simulink model "IndustrialMicrogrid"  (R2023a)
settings: Solver=FixedStepDiscrete  StartTime=0.0  StopTime=10  FixedStep=Ts  RelTol=1e-3
PostLoadFcn:
  | IndustrialMicrogridInputData
  | GfmGridFormingConverterInputParameters
model workspace (MAT data in the model file):
  caseNum = 2
undefined symbols (not defined in the file): base, BESS, DiscIntNeverNeededParam, grid, Grid, gridInverter, machine, microgrid, PV, PVInverter, PVTransformer, scrFactorRg, scrFactorXg, transformer, Ts
libraries: ee_lib x112, eeGeneralControl x104, nesl_utility_internal x64, simulink x56, nesl_utility x37, fl_lib x29, slpidlib x13, eeTransforms x11, eeTotalHarmonicDistorsion x8, eeRmsMeasurement x4, eeSinusoidalMeasurement x4, simulink_extras x2
(part 9 of 14)

== system IndustrialMicrogrid/MG2 PV Plant/(500KWp PV)/PV Inverter A2/PV & Inverter/Measurement1 ==
  u : Inport
  Lead-Lag (Discrete or Continuous) : eeGeneralControl/Lead-Lag (Discrete or Continuous)  T1=0  T2=PV.controllerTSensor  B=inf  A=-inf  init_option=Inherited from block input  x0=0  Ts=Ts
      settings: LibrarySourceBlock=|
      | ee_sl_lib/General Control/Lead-Lag
      | (Discrete or Continuous)
  Out1 : Outport
  wires:
  u/1 -> Lead-Lag (Discrete or Continuous)/1
  Lead-Lag (Discrete or Continuous)/1 -> Out1/1

== system IndustrialMicrogrid/MG2 PV Plant/(500KWp PV)/PV Inverter A2/PV & Inverter/Measurement2 ==
  u : Inport
  Lead-Lag (Discrete or Continuous) : eeGeneralControl/Lead-Lag (Discrete or Continuous)  T1=0  T2=PV.controllerTSensor  B=inf  A=-inf  init_option=Inherited from block input  x0=0  Ts=Ts
      settings: LibrarySourceBlock=|
      | ee_sl_lib/General Control/Lead-Lag
      | (Discrete or Continuous)
  Out1 : Outport
  wires:
  u/1 -> Lead-Lag (Discrete or Continuous)/1
  Lead-Lag (Discrete or Continuous)/1 -> Out1/1

== system IndustrialMicrogrid/MG2 PV Plant/(500KWp PV)/PV Inverter A2/PV & Inverter/P&O MPP ==
  In1 : Inport
  Input : Inport  Port=2
  AND1 : Logic  IconShape=distinctive  AllPortsSameDT=off  OutDataTypeStr=boolean
  Add : Sum
  Compare To Zero1 : simulink/Logic and Bit Operations/Compare To Zero  relop=>=  OutDataTypeStr=boolean
  Compare To Zero2 : simulink/Logic and Bit Operations/Compare To Zero  relop=>=  OutDataTypeStr=boolean
  Constant1 : Constant  Value=PV.mppDv
  NOR : Logic  Operator=NOR  IconShape=distinctive  AllPortsSameDT=off  OutDataTypeStr=boolean
  OR : Logic  Operator=OR  IconShape=distinctive  AllPortsSameDT=off  OutDataTypeStr=boolean
  Subtract5 : Sum  Inputs=-+
  Sum : Sum  Inputs=|+-
  Sum1 : Sum  Inputs=|-+
  Switch4 : Switch  Criteria=u2 ~= 0  SaturateOnIntegerOverflow=off  InputSameDT=off
  Switch5 : Switch  Criteria=u2 > Threshold  SaturateOnIntegerOverflow=off  InputSameDT=off
  Unit Delay : UnitDelay  InitialCondition=2.5e5  SampleTime=PV.mppTs  HasFrameUpgradeWarning=on
  Unit Delay1 : UnitDelay  InitialCondition=1*PVInverter.Vdc  SampleTime=PV.mppTs  HasFrameUpgradeWarning=on
  ZOH/3 : ZeroOrderHold  SampleTime=0.02
  start MPPT Voltage : Constant  Value=PVInverter.Vdc  SampleTime=Ts
  Vmpp : Outport  VectorParamsAs1DForOutWhenUnconnected=off
  wires:
  [Vinc] -> Switch4/1
  ZOH/3/1 -> Vmpp/1
  Unit Delay/1 -> Sum/2
  AND1/1 -> OR/1
  Sum/1 -> Compare To Zero2/1
  Sum1/1 -> Compare To Zero1/1
  Switch4/1 -> ZOH/3/1
  [Vdec] -> Switch4/3
  Subtract5/1 -> [Vdec]  "DEC"
  NOR/1 -> OR/2
  Add/1 -> [Vinc]  "INC"
  Unit Delay1/1 -> Sum1/1
  Input/1 -> Unit Delay1/1, Sum1/2, Switch5/1, Switch5/2
  Constant1/1 -> Subtract5/1, Add/2
  Switch5/1 -> Subtract5/2, Add/1
  In1/1 -> Sum/1, Unit Delay/1
  Compare To Zero2/1 -> AND1/1, NOR/2
  start MPPT Voltage/1 -> Switch5/3
  Compare To Zero1/1 -> AND1/2, NOR/1
  OR/1 -> Switch4/2

== system IndustrialMicrogrid/MG2 PV Plant/(500KWp PV)/PV Inverter A2/PV Controller/Current_controller ==
  id-ref : Inport
  ipvd : Inport  Port=2
  iqref : Inport  Port=3
  iq : Inport  Port=4
  Vd : Inport  Port=5
  Vq : Inport  Port=6
  Constant4 : Constant  Value=0
  Gain1 : Gain  Gain=2*1*pi*60*PVInverter.l/PV.zBase
  Gain2 : Gain  Gain=2*1*pi*60*PVInverter.l/PV.zBase
  Mux1 : Mux  Inputs=3
  PID Controller : slpidlib/PID Controller  Controller=PID  Form=Parallel  TimeDomain=Discrete-time  UseExternalTs=off  SampleTime=-1  IntegratorMethod=Forward Euler  FilterMethod=Forward Euler  ControllerParametersSource=internal  P=PV.controllerKpIc*0.02*2  I=PV.controllerKiIc*0.02*2  UseKiTs=off  D=PV.controllerKd  N=100  UseFilter=off  TunerSelectOption=Transfer Function Based (PID Tuner App)  InitialConditionSource=internal  InitialConditionForIntegrator=-0.023  InitialConditionForFilter=0  DifferentiatorICPrevScaledInput=0  ExternalReset=none  TrackingMode=off  Kt=1  LimitOutput=off  SatLimitsSource=internal  UpperSaturationLimit=1.5  LowerSaturationLimit=-1.5  LinearizeAsGain=on  AntiWindupMode=clamping  Kb=1  LimitIntegrator=off  UpperIntegratorSaturationLimit=1.5  LowerIntegratorSaturationLimit=-1.5  POutMin=[]  POutMax=[]  IOutMin=[]  IOutMax=[]  DOutMin=[]  DOutMax=[]  NOutMin=[]  NOutMax=[]  SumOutMin=[]  SumOutMax=[]  SaturationOutMin=[]  SaturationOutMax=[]  PParamMin=[]  PParamMax=[]  IParamMin=[]  IParamMax=[]  DParamMin=[]  DParamMax=[]  NParamMin=[]  NParamMax=[]  KbParamMin=[]  KbParamMax=[]  KtParamMin=[]  KtParamMax=[]  KbOutMin=[]  KbOutMax=[]  KtOutMin=[]  KtOutMax=[]  IntegratorOutMin=[]  IntegratorOutMax=[]  FilterOutMin=[]  FilterOutMax=[]  SumI1OutMin=[]  SumI1OutMax=[]  SumI2OutMin=[]  SumI2OutMax=[]  SumI3OutMin=[]  SumI3OutMax=[]  SumI4OutMin=[]  SumI4OutMax=[]  SumDOutMin=[]  SumDOutMax=[]  DifferentiatorOutMin=[]  DifferentiatorOutMax=[]  FilterDiffOutCoefMin=[]  FilterDiffOutCoefMax=[]  ReciprocalOutMin=[]  ReciprocalOutMax=[]  SumDenOutMin=[]  SumDenOutMax=[]  SumNumOutMin=[]  SumNumOutMax=[]  DivideOutMin=[]  DivideOutMax=[]  UdiffTsProdOutMin=[]  UdiffTsProdOutMax=[]  NTsProdOutMin=[]  NTsProdOutMax=[]  UintegralTsProdOutMin=[]  UintegralTsProdOutMax=[]  UngainTsProdOutMin=[]  UngainTsProdOutMax=[]  ClampingZeroOutDataTypeStr=Inherit: Inherit via back propagation  ClampingZeroOutMin=[]  ClampingZeroOutMax=[]  FilterDenConstantOutDataTypeStr=Inherit: Inherit via back propagation  FilterDenConstantOutMin=[]  FilterDenConstantOutMax=[]  PCopyOutDataTypeStr=Inherit: Inherit via back propagation  PCopyOutMin=[]  PCopyOutMax=[]  NCopyOutDataTypeStr=Inherit: Inherit via back propagation  NCopyOutMin=[]  NCopyOutMax=[]  IntegratorContinuousStateAttributes=''  IntegratorStateMustResolveToSignalObject=off  IntegratorRTWStateStorageClass=Auto  FilterContinuousStateAttributes=''  FilterStateMustResolveToSignalObject=off  FilterRTWStateStorageClass=Auto  ParallelPVariant=InternalParameters  IdealPVariant=Disabled  IVariant=InternalParameters  DVariant=InternalParameters  IntegratorVariant=Discrete  SatVariant=Disabled  AWVariant=Passthrough  PCopyVariant=Disabled  TRVariant=Disabled  FdbkBlocksVariant=Forward  IdealPFdbkVariant=Disabled  SatFdbkVariant=Disabled  DerivativeFilterVariant=Differentiator  NVariant=Passthrough  NCopyVariant=Disabled_SignalSpec  FilterICVariant=InternalICsDifferentiator  IntegratorICVariant=InternalICs  ExternalResetVariant=Disabled  TRSumVariant=Passthrough  SumFdbkVariant=Disabled  SumVariant=Sum_PID  TsampFilterVariant=InternalTs  TsampNgainVariant=Passthrough  TsampIntegralVariant=Disabled_SignalSpec  ExternalSaturationOutDataTypeStr=Inherit: Same as second input
  PID Controller1 : slpidlib/PID Controller  Controller=PID  Form=Parallel  TimeDomain=Discrete-time  UseExternalTs=off  SampleTime=-1  IntegratorMethod=Forward Euler  FilterMethod=Forward Euler  ControllerParametersSource=internal  P=PV.controllerKpIc*10  I=PV.controllerKiIc*0.2  UseKiTs=off  D=PV.controllerKd  N=100  UseFilter=off  TunerSelectOption=Transfer Function Based (PID Tuner App)  InitialConditionSource=internal  InitialConditionForIntegrator=0.4  InitialConditionForFilter=0  DifferentiatorICPrevScaledInput=0  ExternalReset=none  TrackingMode=off  Kt=1  LimitOutput=off  SatLimitsSource=internal  UpperSaturationLimit=1.5  LowerSaturationLimit=-1.5  LinearizeAsGain=on  AntiWindupMode=clamping  Kb=1  LimitIntegrator=off  UpperIntegratorSaturationLimit=1.5  LowerIntegratorSaturationLimit=-1.5  POutMin=[]  POutMax=[]  IOutMin=[]  IOutMax=[]  DOutMin=[]  DOutMax=[]  NOutMin=[]  NOutMax=[]  SumOutMin=[]  SumOutMax=[]  SaturationOutMin=[]  SaturationOutMax=[]  PParamMin=[]  PParamMax=[]  IParamMin=[]  IParamMax=[]  DParamMin=[]  DParamMax=[]  NParamMin=[]  NParamMax=[]  KbParamMin=[]  KbParamMax=[]  KtParamMin=[]  KtParamMax=[]  KbOutMin=[]  KbOutMax=[]  KtOutMin=[]  KtOutMax=[]  IntegratorOutMin=[]  IntegratorOutMax=[]  FilterOutMin=[]  FilterOutMax=[]  SumI1OutMin=[]  SumI1OutMax=[]  SumI2OutMin=[]  SumI2OutMax=[]  SumI3OutMin=[]  SumI3OutMax=[]  SumI4OutMin=[]  SumI4OutMax=[]  SumDOutMin=[]  SumDOutMax=[]  DifferentiatorOutMin=[]  DifferentiatorOutMax=[]  FilterDiffOutCoefMin=[]  FilterDiffOutCoefMax=[]  ReciprocalOutMin=[]  ReciprocalOutMax=[]  SumDenOutMin=[]  SumDenOutMax=[]  SumNumOutMin=[]  SumNumOutMax=[]  DivideOutMin=[]  DivideOutMax=[]  UdiffTsProdOutMin=[]  UdiffTsProdOutMax=[]  NTsProdOutMin=[]  NTsProdOutMax=[]  UintegralTsProdOutMin=[]  UintegralTsProdOutMax=[]  UngainTsProdOutMin=[]  UngainTsProdOutMax=[]  ClampingZeroOutDataTypeStr=Inherit: Inherit via back propagation  ClampingZeroOutMin=[]  ClampingZeroOutMax=[]  FilterDenConstantOutDataTypeStr=Inherit: Inherit via back propagation  FilterDenConstantOutMin=[]  FilterDenConstantOutMax=[]  PCopyOutDataTypeStr=Inherit: Inherit via back propagation  PCopyOutMin=[]  PCopyOutMax=[]  NCopyOutDataTypeStr=Inherit: Inherit via back propagation  NCopyOutMin=[]  NCopyOutMax=[]  IntegratorContinuousStateAttributes=''  IntegratorStateMustResolveToSignalObject=off  IntegratorRTWStateStorageClass=Auto  FilterContinuousStateAttributes=''  FilterStateMustResolveToSignalObject=off  FilterRTWStateStorageClass=Auto  ParallelPVariant=InternalParameters  IdealPVariant=Disabled  IVariant=InternalParameters  DVariant=InternalParameters  IntegratorVariant=Discrete  SatVariant=Disabled  AWVariant=Passthrough  PCopyVariant=Disabled  TRVariant=Disabled  FdbkBlocksVariant=Forward  IdealPFdbkVariant=Disabled  SatFdbkVariant=Disabled  DerivativeFilterVariant=Differentiator  NVariant=Passthrough  NCopyVariant=Disabled_SignalSpec  FilterICVariant=InternalICsDifferentiator  IntegratorICVariant=InternalICs  ExternalResetVariant=Disabled  TRSumVariant=Passthrough  SumFdbkVariant=Disabled  SumVariant=Sum_PID  TsampFilterVariant=InternalTs  TsampNgainVariant=Passthrough  TsampIntegralVariant=Disabled_SignalSpec  ExternalSaturationOutDataTypeStr=Inherit: Same as second input
  Sum1 : Sum  Inputs=|+-
  Sum3 : Sum  Inputs=|++-
  Sum4 : Sum  Inputs=|+++
  Sum5 : Sum  Inputs=|+-
  Refrence_mdq0 : Outport
  wires:
  ipvd/1 -> Sum1/2, Gain1/1
  id-ref/1 -> Sum1/1
  iq/1 -> Sum5/2, Gain2/1
  iqref/1 -> Sum5/1
  Vd/1 -> Sum3/1
  Vq/1 -> Sum4/2
  Mux1/1 -> Refrence_mdq0/1  "m_dqo"
  Sum4/1 -> Mux1/2
  PID Controller1/1 -> Sum4/1
  Sum5/1 -> PID Controller1/1
  Constant4/1 -> Mux1/3
  Sum1/1 -> PID Controller/1
  Gain1/1 -> Sum4/3
  Gain2/1 -> Sum3/3
  Sum3/1 -> Mux1/1
  PID Controller/1 -> Sum3/2

== system IndustrialMicrogrid/MG2 PV Plant/(500KWp PV)/PV Inverter A2/PV Controller/DC voltage controller & current reference ==
  note: id_ref_generator
  note: iq_ref_generator
  note: Limiter
  Q_ref : Inport
  Vmag : Inport  Port=2
  P_pv : Inport  Port=3
  PV_Mpp_vdc : Inport  Port=4
  PV_vdc : Inport  Port=5
  LVRT.iq : Inport  Port=6
  Constant : Constant
  Constant1 : Constant  Value=PVInverter.iMaxPU
  Current limits : Subsystem
  Subsystem : Subsystem
  Subsystem1 : Subsystem
  Switch : Switch  Criteria=u2 > Threshold  SaturateOnIntegerOverflow=off  InputSameDT=off
  Unit Delay1 : UnitDelay  SampleTime=Ts  HasFrameUpgradeWarning=on
  Unit Delay3 : UnitDelay  SampleTime=Ts  HasFrameUpgradeWarning=on
  iq_ref : Outport
  id_ref : Outport  Port=2
  wires:
  Constant/1 -> Switch/3
  Switch/1 -> Subsystem1/1(Vmag), Subsystem/1(V_mag)
  Vmag/1 -> Switch/1, Switch/2
  LVRT.iq/1 -> Subsystem/3(LVRT.iq)
  [ubiq] -> Subsystem/2(iq_ub)
  [ubid] -> Subsystem1/5(id_ub)
  Subsystem/1(Out1) -> iq_ref/1, [iq_ref]
  PV_vdc/1 -> Subsystem1/4(PV_vdc)
  PV_Mpp_vdc/1 -> Subsystem1/3(PV_Mpp_vdc)
  P_pv/1 -> Subsystem1/2(P_pv)
  Subsystem1/1(Out1) -> id_ref/1, [id_ref]
  Q_ref/1 -> Subsystem/4(Q_ref)
  Unit Delay3/1 -> Current limits/3(idref)
  [id_ref] -> Unit Delay3/1
  Unit Delay1/1 -> Current limits/2(iqref)
  Constant1/1 -> Current limits/1(Imax)
  Current limits/1(iubd) -> [ubid]
  Current limits/2(iubq) -> [ubiq]
  [iq_ref] -> Unit Delay1/1

== system IndustrialMicrogrid/MG2 Primary Substation/BESS and Controller 2/BESS/Grid-Forming Converter Control/Current Limiting ==
  In Bus Element : Inport  PortName=measure  Element=Igd
  In Bus Element1 : Inport  PortName=measure  Element=Igq
  In Bus Element2 : Inport  Port=2  PortName=reactiveControl  Element=Vmd
  In Bus Element4 : Inport  Port=2  PortName=reactiveControl  Element=Vmq
  CurrentLimitingMethod : Subsystem  Variant=on  VariantControlMode=label  VariantControl=Choice  LabelModeActiveChoice=virimp
  Subtract : Sum  Inputs=+-
  Subtract1 : Sum  Inputs=-+
  Out Bus Element : Outport  PortName=currentLimiting  Element=Vmd
  Out Bus Element1 : Outport  PortName=currentLimiting  Element=Vmq
  Out Bus Element2 : Outport  PortName=currentLimiting  Element=Idmax
  Out Bus Element3 : Outport  PortName=currentLimiting  Element=Iqmax
  wires:
  In Bus Element2/1 -> Subtract/1
  In Bus Element1/1 -> CurrentLimitingMethod/2(Igq)
  In Bus Element4/1 -> Subtract1/2
  Subtract/1 -> Out Bus Element/1
  Subtract1/1 -> Out Bus Element1/1
  CurrentLimitingMethod/4(Iqmax) -> Out Bus Element3/1
  In Bus Element/1 -> CurrentLimitingMethod/1(Igd)  "Q"
  CurrentLimitingMethod/3(Idmax) -> Out Bus Element2/1
  CurrentLimitingMethod/1(delVd) -> Subtract/2
  CurrentLimitingMethod/2(delVq) -> Subtract1/1

== system IndustrialMicrogrid/MG2 Primary Substation/BESS and Controller 2/BESS/Grid-Forming Converter Control/Grid Voltage Reactive Power Support ==
  In Bus Element1 : Inport  PortName=measure  Element=Vgd
  In Bus Element3 : Inport  PortName=measure  Element=Vgq
  In Bus Element2 : Inport  PortName=measure  Element=Igd
  In Bus Element4 : Inport  PortName=measure  Element=Igq
  PrefInput : Inport  Port=2
  QrefInput : Inport  Port=3
  Modifying Active Power Reference : Subsystem
  Modifying Reactive Power Reference : Subsystem
  Pref : Outport
  Qref : Outport  Port=2
  wires:
  Modifying Active Power Reference/1(Pref) -> Modifying Reactive Power Reference/4(Pref)
  PrefInput/1 -> Modifying Active Power Reference/1(PrefInput)
  In Bus Element2/1 -> Modifying Active Power Reference/3(Igd)
  In Bus Element4/1 -> Modifying Active Power Reference/4(Igq)
  In Bus Element1/1 -> Modifying Reactive Power Reference/1(Vgd), Modifying Active Power Reference/2(Vd)
  In Bus Element3/1 -> Modifying Reactive Power Reference/2(Vgq)
  QrefInput/1 -> Modifying Reactive Power Reference/3(Qref)
  Modifying Reactive Power Reference/1(PrefNew) -> Pref/1
  Modifying Reactive Power Reference/2(QrefNew) -> Qref/1

== system IndustrialMicrogrid/MG2 Primary Substation/BESS and Controller 2/BESS/Grid-Forming Converter Control/Measurement ==
  Vgabcc : Inport
  Igabc : Inport  Port=2
  Angle : Inport  Port=3
  Frequency Measurement : Subsystem
  Gain1 : Gain  Gain=1/power
  Gain2 : Gain  Gain=1/power
  Gain3 : Gain  Gain=1/(girdLineVoltage*sqrt(2/3))
  Gain4 : Gain  Gain=1/(girdLineVoltage*sqrt(2/3))
  Gain5 : Gain  Gain=1/(power/(sqrt(3)*girdLineVoltage)*sqrt(2))
  Gain6 : Gain  Gain=1/(power/(sqrt(3)*girdLineVoltage)*sqrt(2))
  Power Measurement (Three-Phase) : eePowerMeasurement/Power Measurement (Three-Phase)  LabelModeActiveChoice=Discrete  F=powerFreq  K=[1]  Seq=Positive  Ts=measSampleTime
  abc2dq : Subsystem
  Out Bus Element : Outport  PortName=measure  Element=P
  Out Bus Element1 : Outport  PortName=measure  Element=Q
  Out Bus Element2 : Outport  PortName=measure  Element=Vgd
  Out Bus Element3 : Outport  PortName=measure  Element=Vgq
  Out Bus Element4 : Outport  PortName=measure  Element=Igd
  Out Bus Element5 : Outport  PortName=measure  Element=Igq
  Out Bus Element6 : Outport  PortName=measure  Element=fgrid
  Pmeas : Outport  Port=2
  Qmeas : Outport  Port=3
  fmeas : Outport  Port=4
  wires:
  Vgabcc/1 -> abc2dq/3(Vgabc), Frequency Measurement/1(Vabc), Power Measurement (Three-Phase)/1  "Vabc"
  Angle/1 -> abc2dq/2(Angle)
  Power Measurement (Three-Phase)/1 -> Gain2/1
  Igabc/1 -> abc2dq/1(Igabc), Power Measurement (Three-Phase)/2  "Iabc"
  Power Measurement (Three-Phase)/2 -> Gain1/1
  Gain2/1 -> Pmeas/1, Out Bus Element/1  "Pmeas"
  Gain1/1 -> Qmeas/1, Out Bus Element1/1  "Qmeas"
  abc2dq/1(Vgd) -> Gain4/1
  abc2dq/2(Vgq) -> Gain3/1
  abc2dq/3(Igd) -> Gain5/1
  abc2dq/4(Igq) -> Gain6/1
  Gain3/1 -> Out Bus Element3/1  "Vgq"
  Gain4/1 -> Out Bus Element2/1  "Vgd"
  Gain5/1 -> Out Bus Element4/1  "Igd"
  Gain6/1 -> Out Bus Element5/1  "Igq"
  Frequency Measurement/1(freq) -> Out Bus Element6/1, fmeas/1

== system IndustrialMicrogrid/MG2 Primary Substation/BESS and Controller 2/BESS/Grid-Forming Converter Control/Power Control ==
  note: Reactive Power Control
  note: Active Power Control
  In Bus Element2 : Inport  PortName=measure  Element=P
  In Bus Element1 : Inport  PortName=measure  Element=fgrid
  BusElementIn : Inport  PortName=measure  Element=Vgd
  BusElementIn2 : Inport  PortName=measure  Element=Q
  Pref : Inport  Port=2
  Qref : Inport  Port=3
  Vref : Inport  Port=4
  Fref : Inport  Port=5
  CntrlFlag : Inport  Port=6
  ActivePowerControl : Subsystem  Variant=on  VariantControlMode=label  VariantControl=Choice  LabelModeActiveChoice=vsm
  ReactiveControl : Subsystem
  Scope : Scope
  Out Bus Element : Outport  PortName=reactiveControl  Element=Vmd
  Out Bus Element1 : Outport  PortName=reactiveControl  Element=Vmq
  Out Bus Element6 : Outport  Port=2  PortName=activeControl  Element=angle
  Out Bus Element4 : Outport  Port=2  PortName=activeControl  Element=w
  angle : Outport  Port=3
  wires:
  ActivePowerControl/2(w) -> Out Bus Element4/1
  ActivePowerControl/1(Theta) -> angle/1, Out Bus Element6/1
  ReactiveControl/1(Vmd) -> Out Bus Element/1
  ReactiveControl/2(Vmq) -> Out Bus Element1/1
  Pref/1 -> ActivePowerControl/1(Pref)  "Q"
  Qref/1 -> ReactiveControl/2(Qref)  "Q"
  In Bus Element2/1 -> ActivePowerControl/2(Pmeas)
  In Bus Element1/1 -> ActivePowerControl/5(fgrid)
  Fref/1 -> ActivePowerControl/3(fref)
  CntrlFlag/1 -> [Cntrlflag]
  [Cntrlflag] -> ActivePowerControl/4(cntrlflag)
  Vref/1 -> ReactiveControl/5(Vref)
  [Cntrlflag] -> ReactiveControl/1(CntrlFlag)
  BusElementIn/1 -> Scope/1, ReactiveControl/4(Vgdmeas)
  BusElementIn2/1 -> ReactiveControl/3(Qmeas)

== system IndustrialMicrogrid/MG2 Primary Substation/BESS and Controller 2/BESS/Grid-Forming Converter Control/VoltageCurrentControl ==
  In Bus Element : Inport  PortName=currentLimiting  Element=Vmd
  In Bus Element1 : Inport  PortName=currentLimiting  Element=Vmq
  In Bus Element6 : Inport  PortName=currentLimiting  Element=Idmax
  In Bus Element7 : Inport  PortName=currentLimiting  Element=Iqmax
  Bus Element In6 : Inport  Port=2  PortName=activeControl  Element=w
  Bus Element In1 : Inport  Port=2  PortName=activeControl  Element=angle
  BlackStart : Inport  Port=3
  In Bus Element2 : Inport  Port=4  PortName=measure  Element=Vgd
  In Bus Element3 : Inport  Port=4  PortName=measure  Element=Vgq
  In Bus Element4 : Inport  Port=4  PortName=measure  Element=Igd
  In Bus Element5 : Inport  Port=4  PortName=measure  Element=Igq
  Controller : Subsystem
      settings: PortSchema="{\"entries\":[{\"content\":{\"sides\":[{\"content\":{\"connectorIds\":[\"In1\",\"In2\",\"In3\",\"In4\",\"In5\",\"In6\",\"In7\",\"In8\",\"In9\"]},\"type\":\"ConnectorPlacement.EquallySpacedRectSide\",\"uuid\":\"29d30ab3-0ae0-4ae6-aaee-46c6f5faca9c\"},{\"content\":{\"connectorIds\":[\"Out1\",\"Out2\"],\"side\":\"RIGHT\"},\"type\":\"ConnectorPlacement.EquallySpacedRectSide\",\"uuid\":\"4918c3a7-9f8f-4af5-ac25-a0a0710917b2\"},{\"content\":{\"connectorIds\":[\"In10\"],\"side\":\"TOP\"},\"type\":\"ConnectorPlacement.EquallySpacedRectSide\",\"uuid\":\"c6ee8000-0a39-46c2-b8e8-8b73a56a82d9\"}]},\"type\":\"ConnectorPlacement.EquallySpacedConnector\",\"uuid\":\"193e0bc8-3764-41d1-9278-3938c4a9e9f5\"}],\"packageUris\":[\"http://schema.mathworks.com/mf0/Connector/R2020b\"],\"version\":\"1.0\"}"
  Modulation Signal : Subsystem
  mabc : Outport
  wires:
  Controller/2(Vq) -> Modulation Signal/2(Vq)
  Modulation Signal/1(mabc) -> mabc/1
  Controller/1(Vd) -> Modulation Signal/1(Vd)
  In Bus Element4/1 -> Controller/6(Id)
  In Bus Element5/1 -> Controller/7(Iq)
  In Bus Element6/1 -> Controller/8(Idmax)
  In Bus Element7/1 -> Controller/9(Iqmax)
  In Bus Element2/1 -> Controller/4(Vsd)
  In Bus Element3/1 -> Controller/5(Vsq)
  Bus Element In6/1 -> Controller/1(Angfreq)
  In Bus Element/1 -> Controller/2(Vgdref)
  In Bus Element1/1 -> Controller/3(Vgqref)
  Bus Element In1/1 -> Modulation Signal/3(Angle)
  BlackStart/1 -> Controller/10(BlackStart1)

== system IndustrialMicrogrid/MG2 Primary Substation/Microgrid Controller 2/Black Start/If Action Subsystem/Subsystem ==
  Constant2 : Constant  DisableCoverage=on  Value=-(Controller2BlackStart+Controller2BlackStartDelay)  OutDataTypeStr=Inherit: Inherit via back propagation  SampleTime=Ts
  Digital Clock : DigitalClock  SampleTime=Ts
  Output : Sum  Inputs=|++  InputSameDT=on  SaturateOnIntegerOverflow=on  OutDataTypeStr=Inherit: Same as first input
  Product : Product  DisableCoverage=on  InputSameDT=on  SaturateOnIntegerOverflow=on  OutDataTypeStr=Inherit: Same as first input
  Saturation : Saturate  UpperLimit=Controller2BlackStartVoltageLevel1  LowerLimit=0
  Step : Step  DisableCoverage=on  Time=Controller2BlackStart+Controller2BlackStartDelay  OutDataTypeStr=fixdt('double', 'DataTypeOverride', 'Off')  SampleTime=Ts
  Out1 : Outport
  wires:
  Step/1 -> Product/1
  Output/1 -> Saturation/1
  Product/1 -> Output/1
  Saturation/1 -> Out1/1
  Constant2/1 -> Output/2
  Digital Clock/1 -> Product/2

== system IndustrialMicrogrid/MG2 Primary Substation/Microgrid Controller 2/Black Start/If Action Subsystem/Subsystem1 ==
  Constant2 : Constant  DisableCoverage=on  Value=-(Controller2BlackStart+Controller2BlackStartDelay+Controller2BlackStartDelayLevel2)  OutDataTypeStr=Inherit: Inherit via back propagation  SampleTime=Ts
  Digital Clock : DigitalClock  SampleTime=Ts
  Output : Sum  Inputs=|++  InputSameDT=on  SaturateOnIntegerOverflow=on  OutDataTypeStr=Inherit: Same as first input
  Product : Product  DisableCoverage=on  InputSameDT=on  SaturateOnIntegerOverflow=on  OutDataTypeStr=Inherit: Same as first input
  Saturation : Saturate  UpperLimit=Controller2BlackStartVoltageLevel2  LowerLimit=0
  Step : Step  DisableCoverage=on  Time=Controller2BlackStart+Controller2BlackStartDelay+Controller2BlackStartDelayLevel2  OutDataTypeStr=fixdt('double', 'DataTypeOverride', 'Off')  SampleTime=Ts
  Out1 : Outport
  wires:
  Digital Clock/1 -> Product/2
  Constant2/1 -> Output/2
  Saturation/1 -> Out1/1
  Product/1 -> Output/1
  Output/1 -> Saturation/1
  Step/1 -> Product/1

== system IndustrialMicrogrid/MG2 Primary Substation/Microgrid Controller 2/Black Start/If Action Subsystem/Subsystem2 ==
  Constant2 : Constant  DisableCoverage=on  Value=-(Controller2BlackStart+Controller2BlackStartDelay+Controller2BlackStartDelayLevel2+Controller2BlackStartDelayLevel3)  OutDataTypeStr=Inherit: Inherit via back propagation  SampleTime=Ts
  Digital Clock : DigitalClock  SampleTime=Ts
  Output : Sum  Inputs=|++  InputSameDT=on  SaturateOnIntegerOverflow=on  OutDataTypeStr=Inherit: Same as first input
  Product : Product  DisableCoverage=on  InputSameDT=on  SaturateOnIntegerOverflow=on  OutDataTypeStr=Inherit: Same as first input
  Saturation : Saturate  UpperLimit=Controller2BlackStartVoltageLevel3  LowerLimit=0
  Step : Step  DisableCoverage=on  Time=Controller2BlackStart+Controller2BlackStartDelay+Controller2BlackStartDelayLevel2+Controller2BlackStartDelayLevel3  OutDataTypeStr=fixdt('double', 'DataTypeOverride', 'Off')  SampleTime=Ts
  Out1 : Outport
  wires:
  Step/1 -> Product/1
  Output/1 -> Saturation/1
  Product/1 -> Output/1
  Saturation/1 -> Out1/1
  Constant2/1 -> Output/2
  Digital Clock/1 -> Product/2

== system IndustrialMicrogrid/MG2 Primary Substation/Microgrid Controller 2/PLL /PLL/Subsystem ==
  In : Inport
  Bias : Bias  Bias=180  SaturateOnIntegerOverflow=off
  Bias1 : Bias  Bias=-180  SaturateOnIntegerOverflow=off
  Constant : Constant  Value=grid.frequency
  Constant1 : Constant  Value=360
  Data Type Conversion Inherited : simulink/Signal Attributes/Data Type Conversion Inherited  ConvertRealWorld=Real World Value  DoSatur=off
  Digital Clock : DigitalClock  SampleTime=Ts
  Mod : Math  Operator=mod
  Product : Product
  Sum : Sum  Inputs=+-  OutDataTypeStr=Inherit: Same as first input
  gain : Gain  Gain=2*pi
  rad2deg : Gain  Gain=180/pi
  Out : Outport
  wires:
  Bias1/1 -> Out/1
  Product/1 -> Sum/2
  In/1 -> Sum/1
  gain/1 -> Product/1
  Constant/1 -> gain/1
  Bias/1 -> Mod/1
  Mod/1 -> Bias1/1
  Digital Clock/1 -> Product/2
  Constant1/1 -> Data Type Conversion Inherited/2
  rad2deg/1 -> Data Type Conversion Inherited/1, Bias/1
  Sum/1 -> rad2deg/1
  Data Type Conversion Inherited/1 -> Mod/2

== system IndustrialMicrogrid/MG2 Primary Substation/Microgrid Controller 2/PLL /PLL1/Subsystem ==
  In : Inport
  Bias : Bias  Bias=180  SaturateOnIntegerOverflow=off
  Bias1 : Bias  Bias=-180  SaturateOnIntegerOverflow=off
  Constant : Constant  Value=grid.frequency
  Constant1 : Constant  Value=360
  Data Type Conversion Inherited : simulink/Signal Attributes/Data Type Conversion Inherited  ConvertRealWorld=Real World Value  DoSatur=off
  Digital Clock : DigitalClock  SampleTime=Ts
  Mod : Math  Operator=mod
  Product : Product
  Sum : Sum  Inputs=+-  OutDataTypeStr=Inherit: Same as first input
  gain : Gain  Gain=2*pi
  rad2deg : Gain  Gain=180/pi
  Out : Outport
  wires:
  Data Type Conversion Inherited/1 -> Mod/2
  Sum/1 -> rad2deg/1
  rad2deg/1 -> Bias/1, Data Type Conversion Inherited/1
  Constant1/1 -> Data Type Conversion Inherited/2
  Digital Clock/1 -> Product/2
  Mod/1 -> Bias1/1
  Bias/1 -> Mod/1
  Constant/1 -> gain/1
  gain/1 -> Product/1
  In/1 -> Sum/1
  Product/1 -> Sum/2
  Bias1/1 -> Out/1

== system IndustrialMicrogrid/MG2 Primary Substation/Microgrid Controller 2/Planned Island/Control for Zero Powerflow1/Planned Island Time Delay ==
  In1 : Inport
  In2 : Inport  Port=2
  Cast To Double : DataTypeConversion  OutDataTypeStr=double  SaturateOnIntegerOverflow=off  RndMeth=Floor
  Constant3 : Constant  Value=0
  Delay1 : Delay  DelayLength=500  SampleTime=Ts
  Delay2 : Delay  DelayLength=PlannedIslandDelay  InitialCondition=0  SampleTime=Ts*5
  Monostable Flip-Flop : eeGeneralControl/Monostable Flip-Flop  VariantControl=Variant1  LabelModeActiveChoice=Discrete  ChangeType=Rising edge  x0=0  Td=100  Ts=Ts
      settings: LibrarySourceBlock=ee_sl_lib/General Control/Monostable Flip-Flop
  Switch : Switch  Criteria=u2 > Threshold  Threshold=0.5  SaturateOnIntegerOverflow=off  InputSameDT=off
  MGController : Outport
  wires:
  In2/1 -> Delay1/1
  In1/1 -> Switch/1
  Monostable Flip-Flop/1 -> Cast To Double/1
  Delay2/1 -> MGController/1
  Delay1/1 -> Switch/2
  Constant3/1 -> Switch/3
  Cast To Double/1 -> Delay2/1
  Switch/1 -> Monostable Flip-Flop/1

== system IndustrialMicrogrid/MG2 Primary Substation/Microgrid Controller 2/Planned Island/Control for Zero Powerflow1/Subsystem ==
  AVTIVE POWER ERROR : Inport
  AND : Logic  IconShape=distinctive  AllPortsSameDT=off  OutDataTypeStr=boolean
  Abs : Abs  SaturateOnIntegerOverflow=off
  Constant : Constant  Value=ZeroActivePowerThreshold  SampleTime=-1
  Delay : Delay  DelayLength=1000  SampleTime=Ts
  Relational Operator : RelationalOperator  Operator=<=  OutDataTypeStr=boolean  RndMeth=Simplest  InputSameDT=off
  Out1 : Outport
  wires:
  Delay/1 -> AND/2
  Constant/1 -> Relational Operator/2
  Relational Operator/1 -> AND/1, Delay/1
  AND/1 -> Out1/1
  AVTIVE POWER ERROR/1 -> Abs/1
  Abs/1 -> Relational Operator/1

== system IndustrialMicrogrid/MG2 Primary Substation/Microgrid Controller 2/Planned Island/Control for Zero Powerflow1/Subsystem1 ==
  REACTIVEPOWER ERROR : Inport
  AND : Logic  IconShape=distinctive  AllPortsSameDT=off  OutDataTypeStr=boolean
  Abs : Abs  SaturateOnIntegerOverflow=off
  Constant2 : Constant  Value=ZeroReactivePowerThreshold
  Delay : Delay  DelayLength=1000  SampleTime=Ts
  Relational Operator2 : RelationalOperator  Operator=<=  OutDataTypeStr=boolean  RndMeth=Simplest  InputSameDT=off
  Out1 : Outport
  wires:
  Delay/1 -> AND/2
  REACTIVEPOWER ERROR/1 -> Abs/1
  Relational Operator2/1 -> Delay/1, AND/1
  Constant2/1 -> Relational Operator2/2
  AND/1 -> Out1/1
  Abs/1 -> Relational Operator2/1

== system IndustrialMicrogrid/MG2 Primary Substation/Microgrid Controller 2/Resynchronization/Frequency and voltage matching/Resynchronization Time Delay ==
  In1 : Inport
  In2 : Inport  Port=2
  Cast To Double : DataTypeConversion  OutDataTypeStr=double  SaturateOnIntegerOverflow=off  RndMeth=Floor
  Constant3 : Constant  Value=0
  Delay1 : Delay  DelayLength=500  SampleTime=Ts
  Delay2 : Delay  DelayLength=ResynchDelay  InitialCondition=0  SampleTime=Ts*5
  Monostable Flip-Flop : eeGeneralControl/Monostable Flip-Flop  VariantControl=Variant1  LabelModeActiveChoice=Discrete  ChangeType=Rising edge  x0=0  Td=100  Ts=Ts
      settings: LibrarySourceBlock=ee_sl_lib/General Control/Monostable Flip-Flop
  Switch : Switch  Criteria=u2 > Threshold  Threshold=0.5  SaturateOnIntegerOverflow=off  InputSameDT=off
  MGController : Outport
  wires:
  Switch/1 -> Monostable Flip-Flop/1
  Cast To Double/1 -> Delay2/1
  Constant3/1 -> Switch/3
  Delay1/1 -> Switch/2
  Delay2/1 -> MGController/1
  Monostable Flip-Flop/1 -> Cast To Double/1
  In1/1 -> Switch/1
  In2/1 -> Delay1/1

== system IndustrialMicrogrid/MG2 Primary Substation/Microgrid Controller 2/Resynchronization/Frequency and voltage matching/Subsystem ==
  FREQUENCY ERROR : Inport
  AND : Logic  IconShape=distinctive  AllPortsSameDT=off  OutDataTypeStr=boolean
  Abs : Abs  SaturateOnIntegerOverflow=off
  Constant : Constant  Value=FrequencyThreshold  SampleTime=-1
  Delay : Delay  DelayLength=1000  SampleTime=Ts
  Relational Operator : RelationalOperator  Operator=<=  OutDataTypeStr=boolean  RndMeth=Simplest  InputSameDT=off
  Out1 : Outport
  wires:
  Delay/1 -> AND/2
  Constant/1 -> Relational Operator/2
  Relational Operator/1 -> AND/1, Delay/1
  AND/1 -> Out1/1
  FREQUENCY ERROR/1 -> Abs/1
  Abs/1 -> Relational Operator/1

== system IndustrialMicrogrid/MG2 Primary Substation/Microgrid Controller 2/Resynchronization/Frequency and voltage matching/Subsystem1 ==
  ANGLE ERROR : Inport
  AND : Logic  IconShape=distinctive  AllPortsSameDT=off  OutDataTypeStr=boolean
  Abs : Abs  SaturateOnIntegerOverflow=off
  Constant1 : Constant  Value=AngleThreshold
  Delay : Delay  DelayLength=1000  SampleTime=Ts
  Relational Operator : RelationalOperator  Operator=<=  OutDataTypeStr=boolean  RndMeth=Simplest  InputSameDT=off
  Out1 : Outport
  wires:
  ANGLE ERROR/1 -> Abs/1
  AND/1 -> Out1/1
  Relational Operator/1 -> Delay/1, AND/1
  Constant1/1 -> Relational Operator/2
  Delay/1 -> AND/2
  Abs/1 -> Relational Operator/1

== system IndustrialMicrogrid/MG2 Primary Substation/Microgrid Controller 2/Resynchronization/Frequency and voltage matching/Subsystem2 ==
  VOLTAGE ERROR : Inport
  AND : Logic  IconShape=distinctive  AllPortsSameDT=off  OutDataTypeStr=boolean
  Abs : Abs  SaturateOnIntegerOverflow=off
  Constant2 : Constant  Value=VoltageThreshold
  Delay : Delay  DelayLength=1000  SampleTime=Ts
  Relational Operator : RelationalOperator  Operator=<=  OutDataTypeStr=boolean  RndMeth=Simplest  InputSameDT=off
  Out1 : Outport
  wires:
  Delay/1 -> AND/2
  Constant2/1 -> Relational Operator/2
  Relational Operator/1 -> AND/1, Delay/1
  AND/1 -> Out1/1
  VOLTAGE ERROR/1 -> Abs/1
  Abs/1 -> Relational Operator/1

== system IndustrialMicrogrid/MG2 Primary Substation/Microgrid Controller 2/Resynchronization/Frequency and voltage matching/Synch Voltage ==
  MicrogridController : Inport
  ControlRoom : Inport  Port=2
  u : Inport  Port=3
  Resynch : Inport  Port=4
  Gain1 : Gain  Gain=microgrid.KDroop
  Logical Operator1 : Logic  Operator=NOT  AllPortsSameDT=off  OutDataTypeStr=boolean
  Low-Pass Filter (Discrete or Continuous) : eeGeneralControl/Low-Pass Filter (Discrete or Continuous)  K=1  T=0.08  B=inf  A=-inf  init_option=Specify as parameter  x0=0  Ts=5*Ts
  Sample and Hold : spsSampleandHoldLib/Sample and Hold  ic=0  Ts=Ts
  Subsystem2 : Subsystem
  Sum4 : Sum  Inputs=+-
  Out1 : Outport
  wires:
  Low-Pass Filter (Discrete or Continuous)/1 -> Gain1/1
  Resynch/1 -> Logical Operator1/1
  Sample and Hold/1 -> Sum4/1
  Gain1/1 -> Sum4/2
  Logical Operator1/1 -> Sample and Hold/2
  MicrogridController/1 -> Subsystem2/1(MicrogridController)
  Subsystem2/1(Out1) -> Sample and Hold/1
  Sum4/1 -> Out1/1
  ControlRoom/1 -> Subsystem2/2(ControlRoom)
  u/1 -> Low-Pass Filter (Discrete or Continuous)/1

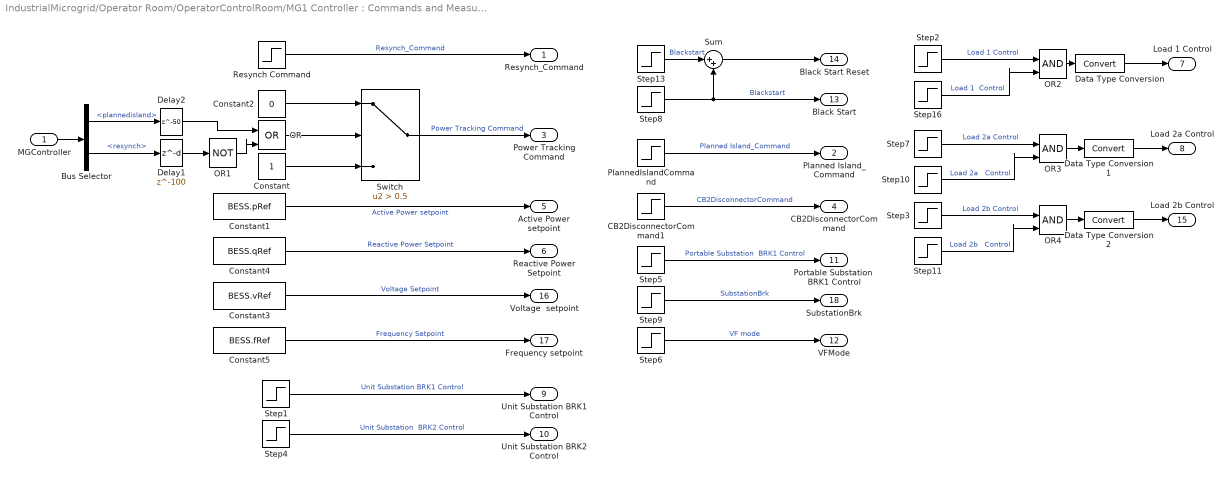
== system IndustrialMicrogrid/Operator Room/OperatorControlRoom/MG1 Controller : Commands and Measurements/Microgrid Controller 1 : Commands and Measurements/Command and setpoints ==
  MGController : Inport
  Bus Selector : BusSelector  OutputSignals=Controller.IslandMGController.MGPlannedIsland.plannedisland,Controller.ResynchMGController.MGResynch.resynch
  CB2DisconnectorCommand1 : Step  Time=microgrid.controller1PCCBrk  SampleTime=Ts
  Constant : Constant
  Constant1 : Constant  Value=BESS.pRef  SampleTime=-1
  Constant2 : Constant  Value=0
  Constant3 : Constant  Value=BESS.vRef  SampleTime=-1
  Constant4 : Constant  Value=BESS.qRef  SampleTime=-1
  Constant5 : Constant  Value=BESS.fRef  SampleTime=-1
  Data Type Conversion : DataTypeConversion  SaturateOnIntegerOverflow=off  RndMeth=Floor
  Data Type Conversion1 : DataTypeConversion  SaturateOnIntegerOverflow=off  RndMeth=Floor
  Data Type Conversion2 : DataTypeConversion  SaturateOnIntegerOverflow=off  RndMeth=Floor
  Delay1 : Delay  DelayLength=100  InitialCondition=0  SampleTime=Ts*45*1000
  Delay2 : Delay  DelayLength=50  InitialCondition=0  SampleTime=Ts*45
  OR : Logic  Operator=OR  IconShape=distinctive  AllPortsSameDT=off  OutDataTypeStr=boolean
  OR1 : Logic  Operator=NOT  IconShape=distinctive  AllPortsSameDT=off  OutDataTypeStr=boolean
  OR2 : Logic  IconShape=distinctive  AllPortsSameDT=off  OutDataTypeStr=boolean
  OR3 : Logic  IconShape=distinctive  AllPortsSameDT=off  OutDataTypeStr=boolean
  OR4 : Logic  IconShape=distinctive  AllPortsSameDT=off  OutDataTypeStr=boolean
  PlannedIslandCommand : Step  Time=microgrid.controller1PlannedIsland  SampleTime=Ts
  Resynch Command : Step  Time=microgrid.controller1Resynch  SampleTime=Ts
  Step1 : Step  Time=microgrid.controller1UnitSubstationBrk1  SampleTime=Ts
  Step10 : Step  Time=microgrid.controller1BlackStart+microgrid.controller1BlackStartDelay+microgrid.controller1BlackStartBlockLoad1PickUp1+microgrid.controller1BlackStartBlockLoad1PickUp2  Before=1  After=0  SampleTime=Ts
  Step11 : Step  Time=microgrid.controller1BlackStart+microgrid.controller1BlackStartDelay+microgrid.controller2BlackStartBlockLoad1PickUp1+microgrid.controller1BlackStartBlockLoad1PickUp2+microgrid.controller1BlackStartBlockLoad1PickUp3  Before=1  SampleTime=Ts
  Step13 : Step  Time=microgrid.controller1BlackStart+microgrid.controller1BlackStartDelay  After=-1  SampleTime=Ts
  Step16 : Step  Time=microgrid.controller1BlackStart+microgrid.controller1BlackStartDelay+microgrid.controller1BlackStartBlockLoad1PickUp1  Before=1  After=0  SampleTime=Ts
  Step2 : Step  Time=microgrid.controller1Load1Control  Before=1  After=0  SampleTime=Ts
  Step3 : Step  Time=microgrid.controller1Load2Control  Before=1  After=0  SampleTime=Ts
  Step4 : Step  Time=microgrid.controller1UnitSubstationBrk2  SampleTime=Ts
  Step5 : Step  Time=microgrid.controller1PortableSubstationBrk  Before=1  After=0  SampleTime=Ts
  Step6 : Step  Time=microgrid.controller1VFMode  SampleTime=Ts
  Step7 : Step  Time=microgrid.controller1Load2Control  Before=1  After=0  SampleTime=Ts
  Step8 : Step  Time=microgrid.controller1BlackStart  SampleTime=Ts
  Step9 : Step  Time=microgrid.controller1SubstationBrk  SampleTime=Ts
  Sum : Sum  Inputs=|++
  Switch : Switch  Criteria=u2 > Threshold  Threshold=0.5  SaturateOnIntegerOverflow=off  InputSameDT=off
  Resynch_Command : Outport
  Planned Island_Command : Outport  Port=2
  Power Tracking Command : Outport  Port=3
  CB2DisconnectorCommand : Outport  Port=4
  Active Power setpoint : Outport  Port=5
  Reactive Power Setpoint : Outport  Port=6
  Load 1 Control : Outport  Port=7
  Load 2a Control : Outport  Port=8
  Unit Substation BRK1 Control : Outport  Port=9
  Unit Substation BRK2 Control : Outport  Port=10
  Portable Substation  BRK1 Control : Outport  Port=11
  VFMode : Outport  Port=12
  Black Start : Outport  Port=13
  Black Start Reset : Outport  Port=14
  Load 2b Control : Outport  Port=15
  Voltage  setpoint : Outport  Port=16
  Frequency setpoint : Outport  Port=17
  SubstationBrk : Outport  Port=18
  wires:
  PlannedIslandCommand/1 -> Planned Island_Command/1  "Planned Island_Command"
  Bus Selector/1 -> Delay2/1  "<plannedisland>"
  Switch/1 -> Power Tracking Command/1  "Power Tracking Command"
  Resynch Command/1 -> Resynch_Command/1  "Resynch_Command"
  Delay2/1 -> OR/1
  Bus Selector/2 -> Delay1/1  "<resynch>"
  Constant2/1 -> Switch/1
  OR/1 -> Switch/2
  Constant/1 -> Switch/3
  CB2DisconnectorCommand1/1 -> CB2DisconnectorCommand/1  "CB2DisconnectorCommand"
  Constant1/1 -> Active Power setpoint/1  "Active Power setpoint"
  OR1/1 -> OR/2
  Delay1/1 -> OR1/1
  MGController/1 -> Bus Selector/1
  Constant4/1 -> Reactive Power Setpoint/1  "Reactive Power Setpoint"
  Step1/1 -> Unit Substation BRK1 Control/1  "Unit Substation BRK1 Control"
  Step4/1 -> Unit Substation BRK2 Control/1  "Unit Substation  BRK2 Control"
  Step5/1 -> Portable Substation  BRK1 Control/1  "Portable Substation  BRK1 Control"
  Step6/1 -> VFMode/1  "VF mode"
  Step13/1 -> Sum/1  "Blackstart"
  Step8/1 -> Sum/2, Black Start/1  "Blackstart"
  Sum/1 -> Black Start Reset/1
  Data Type Conversion/1 -> Load 1 Control/1
  OR3/1 -> Data Type Conversion1/1
  Step11/1 -> OR4/2  "Load 2b   Control"
  OR2/1 -> Data Type Conversion/1
  Step10/1 -> OR3/2  "Load 2a   Control"
  Step7/1 -> OR3/1  "Load 2a Control"
  Step16/1 -> OR2/2  "Load 1  Control"
  Step3/1 -> OR4/1  "Load 2b Control"
  OR4/1 -> Data Type Conversion2/1
  Data Type Conversion1/1 -> Load 2a Control/1
  Data Type Conversion2/1 -> Load 2b Control/1
  Step2/1 -> OR2/1  "Load 1 Control"
  Constant3/1 -> Voltage  setpoint/1  "Voltage Setpoint"
  Constant5/1 -> Frequency setpoint/1  "Frequency Setpoint"
  Step9/1 -> SubstationBrk/1  "SubstationBrk"

== system IndustrialMicrogrid/Operator Room/OperatorControlRoom/MG1 Controller : Commands and Measurements/Microgrid Controller 1 : Commands and Measurements/Measurements and visualizations  ==
  In Bus Element25 : Inport  PortName=mLoad  Element=active power
  In Bus Element17 : Inport  PortName=mLoad  Element=voltageRMS
  In Bus Element20 : Inport  PortName=mLoad  Element=current
  In Bus Element26 : Inport  PortName=mLoad  Element=reactive power
  In Bus Element22 : Inport  PortName=mLoad  Element=voltage
  In Bus Element5 : Inport  Port=2  PortName=MGController  Element=Controller.ResynchMGController.PCC measurments.Grid.angle
  In Bus Element3 : Inport  Port=2  PortName=MGController  Element=Controller.ResynchMGController.PCC measurments.Grid.frequency
  In Bus Element4 : Inport  Port=2  PortName=MGController  Element=Controller.ResynchMGController.PCC measurments.Grid.voltage
  In Bus Element8 : Inport  Port=2  PortName=MGController  Element=Controller.ResynchMGController.PCC measurments.Island.voltage
  In Bus Element7 : Inport  Port=2  PortName=MGController  Element=Controller.ResynchMGController.PCC measurments.Island.angle
  In Bus Element6 : Inport  Port=2  PortName=MGController  Element=Controller.ResynchMGController.PCC measurments.Island.frequency
  In Bus Element18 : Inport  Port=2  PortName=MGController  Element=Controller.ResynchMGController.PCC measurments.PCC.mPCC.current
  In Bus Element19 : Inport  Port=2  PortName=MGController  Element=Controller.ResynchMGController.PCC measurments.PCC.mPCC.voltage
  In Bus Element27 : Inport  Port=2  PortName=MGController  Element=Controller.ResynchMGController.PCC measurments.PCC.mPCC.activepower
  In Bus Element28 : Inport  Port=2  PortName=MGController  Element=Controller.ResynchMGController.PCC measurments.PCC.mPCC.reactivepower
  In Bus Element10 : Inport  Port=2  PortName=MGController  Element=Controller.ResynchMGController.MGResynch.voltagemagerror
  In Bus Element11 : Inport  Port=2  PortName=MGController  Element=Controller.ResynchMGController.MGResynch.phaseerror
  In Bus Element9 : Inport  Port=2  PortName=MGController  Element=Controller.ResynchMGController.MGResynch.frequencyerror
  In Bus Element : Inport  Port=2  PortName=MGController  Element=Controller.ResynchMGController.MGResynch.resynch
  In Bus Element12 : Inport  Port=2  PortName=MGController  Element=Controller.IslandMGController.MGPlannedIsland.plannedisland
  In Bus Element14 : Inport  Port=2  PortName=MGController  Element=BESS.voltage
  In Bus Element15 : Inport  Port=2  PortName=MGController  Element=BESS.current
  In Bus Element29 : Inport  Port=2  PortName=MGController  Element=BESS.active power
  In Bus Element30 : Inport  Port=2  PortName=MGController  Element=BESS.reactive power
  Resynch : Inport  Port=3
  PlannedIslandCmd : Inport  Port=4
  Power Tracking Command : Inport  Port=5
  "BESS, PV and Load Measurements" : Subsystem
  Resynchronization and Planned Islanding : Subsystem
  Active Power : Outport
  Reactive Power : Outport  Port=2
  wires:
  In Bus Element3/1 -> Resynchronization and Planned Islanding/1(Grid Frequency)  "Grid Frequency"
  In Bus Element6/1 -> Resynchronization and Planned Islanding/2(Island Frequency)  "Island Frequency"
  Resynch/1 -> Resynchronization and Planned Islanding/3(Resynch)  "Resynch Command"
  In Bus Element5/1 -> Resynchronization and Planned Islanding/4(Grid Angle)  "Grid Angle"
  In Bus Element7/1 -> Resynchronization and Planned Islanding/5(Island Angle)  "Island Angle"
  In Bus Element/1 -> Resynchronization and Planned Islanding/6(Resynchronization)  "Resynchronization"
  In Bus Element4/1 -> Resynchronization and Planned Islanding/7(Grid Voltage)  "Grid Voltage"
  In Bus Element18/1 -> Resynchronization and Planned Islanding/8(Grid Current)  "Grid Current"
  In Bus Element8/1 -> Resynchronization and Planned Islanding/9(Island Voltage)  "Island Voltage"
  In Bus Element9/1 -> Resynchronization and Planned Islanding/10(Frequency Error)  "Frequency Error"
  In Bus Element19/1 -> Resynchronization and Planned Islanding/11(Grid Voltage1)  "Grid Voltage"
  In Bus Element11/1 -> Resynchronization and Planned Islanding/12(Phase Angle Error)  "Phase Angle Error"
  In Bus Element10/1 -> Resynchronization and Planned Islanding/13(Voltage Error)  "Voltage Error"
  In Bus Element27/1 -> "BESS, PV and Load Measurements"/1(Grid Active Power)  "Grid Active Power"
  In Bus Element15/1 -> "BESS, PV and Load Measurements"/5(BESS Current)  "BESS Current"
  In Bus Element25/1 -> "BESS, PV and Load Measurements"/6(Load Active Power)  "Load Active Power"
  In Bus Element28/1 -> "BESS, PV and Load Measurements"/2(Grid Reactive Power)  "Grid Reactive Power"
  In Bus Element30/1 -> "BESS, PV and Load Measurements"/7(BESS Reactive Power)  "BESS Reactive Power"
  In Bus Element26/1 -> "BESS, PV and Load Measurements"/8(Load Reactive Power)  "Load Reactive Power"
  In Bus Element20/1 -> "BESS, PV and Load Measurements"/9(Load Current(p.u.))  "Load Current(p.u.)"
  In Bus Element22/1 -> "BESS, PV and Load Measurements"/10(Load Voltage (p.u.))  "Load Voltage (p.u.)"
  In Bus Element17/1 -> "BESS, PV and Load Measurements"/11(Load Voltage RMS (p.u.))  "Load Voltage RMS (p.u.)"
  In Bus Element29/1 -> "BESS, PV and Load Measurements"/3(BESS Active Power)  "BESS Active Power"
  In Bus Element14/1 -> "BESS, PV and Load Measurements"/4(BESS Voltage)  "BESS Voltage"
  PlannedIslandCmd/1 -> Resynchronization and Planned Islanding/14(PlannedIslandCommand)
  In Bus Element12/1 -> Resynchronization and Planned Islanding/15(PlannedIsland)  "Voltage Error"
  Power Tracking Command/1 -> Resynchronization and Planned Islanding/16(Power Tracking Command)
  "BESS, PV and Load Measurements"/1(Active Power) -> Active Power/1
  "BESS, PV and Load Measurements"/2(Reactive Power) -> Reactive Power/1

== system IndustrialMicrogrid/Operator Room/OperatorControlRoom/MG1 Controller : Commands and Measurements/Microgrid Controller 1 : Commands and Measurements/Monitoring of system performance ==
  Active and Reactive Power : Inport
  mLoad3 : Inport  Port=2
  Tieline : Inport  Port=3
  In Bus Element1 : Inport  Port=4  PortName=mLoad  Element=active power
  In Bus Element4 : Inport  Port=4  PortName=mLoad  Element=voltage
  In Bus Element5 : Inport  Port=4  PortName=mLoad  Element=voltageRMS
  In Bus Element7 : Inport  Port=4  PortName=mLoad  Element=current
  In Bus Element9 : Inport  Port=4  PortName=mLoad  Element=currentRMS
  In Bus Element10 : Inport  Port=5  PortName=MGController  Element=Controller.IslandMGController.PCC measurments.PCC.mPCC.current
  In Bus Element6 : Inport  Port=5  PortName=MGController  Element=Controller.ResynchMGController.PCC measurments.Island.frequency
  In Bus Element8 : Inport  Port=5  PortName=MGController  Element=Controller.ResynchMGController.PCC measurments.Island.voltage
  In Bus Element2 : Inport  Port=5  PortName=MGController  Element=Controller.ResynchMGController.PCC measurments.PCC.mPCC.voltage
  "Load " : Subsystem
  Microgrid : Subsystem
  Subsystem : Subsystem
  THD : Subsystem
  wires:
  In Bus Element4/1 -> THD/1(mLoad)
  In Bus Element7/1 -> THD/2(In2)
  In Bus Element2/1 -> THD/3(MGController)
  In Bus Element10/1 -> THD/4(In4)
  In Bus Element6/1 -> Microgrid/1(Frequency)
  In Bus Element8/1 -> Microgrid/2(Voltage)
  In Bus Element5/1 -> "Load "/1(In1)
  In Bus Element9/1 -> "Load "/2(In2)
  In Bus Element1/1 -> "Load "/3(In3)
  Active and Reactive Power/1 -> Subsystem/1(Active and Reactive Power)
  Tieline/1 -> Subsystem/2(mtieline1)
  mLoad3/1 -> Subsystem/3(mLoad3)
